simulink model "Template10HzUno"  (R2018b)
settings: Solver=ode4  StartTime=0.0  StopTime=7200  FixedStep=0.1  RelTol=1e-3  EnableMultiTasking=on
settings Model: EnablePacing=on  ExtModeTrigDuration=2  Creator=user  LastModifiedBy=auralius
settings OptimizationCC: EnhancedBackFolding=on  PassReuseOutputArgsAs=Individual arguments  MaxStackSize=64  OptimizeBlockOrder=speed  DifferentSizesBufferReuse=on  OptimizationCustomize=off
settings DebuggingCC: ParameterTunabilityLossMsg=error  LibraryContextMissingDiagnostic=none
settings HardwareCC: ProdBitPerInt=16  ProdBitPerPointer=16  ProdBitPerSizeT=16  ProdBitPerPtrDiffT=16  ProdLargestAtomicFloat=None  ProdWordSize=8  ProdHWDeviceType=Atmel->AVR
settings SFSimCC: SimUseLocalCustomCode=off  MATLABDynamicMemAlloc=off
settings SFSimCC: SimCustomTerminator=|
  | analogWrite(9, 0);
  | analogWrite(10, 0);
  | delay(1);
settings RTWCC: SystemTargetFile=ert.tlc  HardwareBoard=Arduino Uno  TemplateMakefile=ert_default_tmf  GenerateReport=on  RTWUseLocalCustomCode=off  Toolchain=Arduino AVR  BuildConfiguration=Faster Runs  IncludeHyperlinkInReport=on  LaunchReport=on  GenerateTraceInfo=on  GenerateTraceReport=on  GenerateTraceReportSl=on  GenerateTraceReportSf=on  GenerateTraceReportEml=on
settings CodeAppCC: ForceParamTrailComments=on  IgnoreCustomStorageClasses=off  OperatorAnnotations=on  SimulinkDataObjDesc=on  SFDataObjDesc=on  InsertBlockDesc=on
settings ERTTargetCC: SupportContinuousTime=on  SupportVariableSizeSignals=on  ExtMode=on  ExtModeMexArgs='127.0.0.1' 0 17725

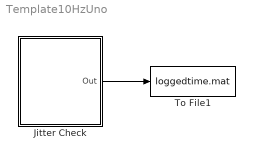
== system Template10HzUno ==
  Jitter Check : Subsystem
  To File1 : ToFile  Filename=loggedtime.mat  MatrixName=ts
  wires:
  Jitter Check/1(Out) -> To File1/1

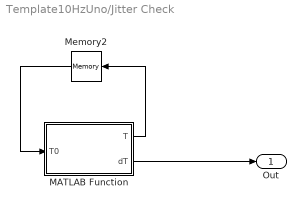
== system Template10HzUno/Jitter Check ==
  MATLAB Function : MATLAB Function  TreatAsAtomicUnit=on
  Memory2 : Memory  InheritSampleTime=on
  Out : Outport
  wires:
  MATLAB Function/2(dT) -> Out/1
  Memory2/1 -> MATLAB Function/1(T0)
  MATLAB Function/1(T) -> Memory2/1

== matlab function Template10HzUno/Jitter Check/MATLAB Function ==
  data: T output; T0 input; dT output
function [T, dT]= get_time(T0)

coder.extrinsic('now');
coder.extrinsic('datevec');

T = 0;
dT = 0;

[~, ~, ~, ~, ~, T] = datevec(now);

if T>T0
    dT = T-T0;
else
    dT = T-T0+60;
end

end
